simulink model "fxpdemo_sfun_user_prodsum"  (Simulink 7.6)
settings: Solver=FixedStepDiscrete  StartTime=0.0  StopTime=0.2  FixedStep=0.001  RelTol=1e-3
libraries: simulink x3
Description:
  | Fixed-Point S-Functions: Product and Sum
  | 
  | This model exercises a custom C language S-function written to compute a fixed-point
  | "product and sum" operation.  To see the source code for the S-function, use the right-click context menu to
  | select "Look Under Mask".  When the dialog box appears, press the Edit button.
settings Model: Creator=The MathWorks Inc.  ExtModeAutoUpdateStatusClock=off
settings DataIOCC: SignalLoggingName=sigsOut
settings OptimizationCC: InlineParams=on  InitFltsAndDblsToZero=on
settings DebuggingCC: SaveWithParameterizedLinksMsg=none  SignalResolutionControl=TryResolveAllWithWarning  SolverPrmCheckMsg=none  MultiTaskDSMMsg=warning  MultiTaskCondExecSysMsg=none  ParameterPrecisionLossMsg=none  StrictBusMsg=None
settings HardwareCC: TargetUnknown=on
settings RTWCC: GenerateReport=on  IncludeERTFirstTime=on
settings GRTTargetCC: TargetFcnLib=ansi_tfl_tmw.mat

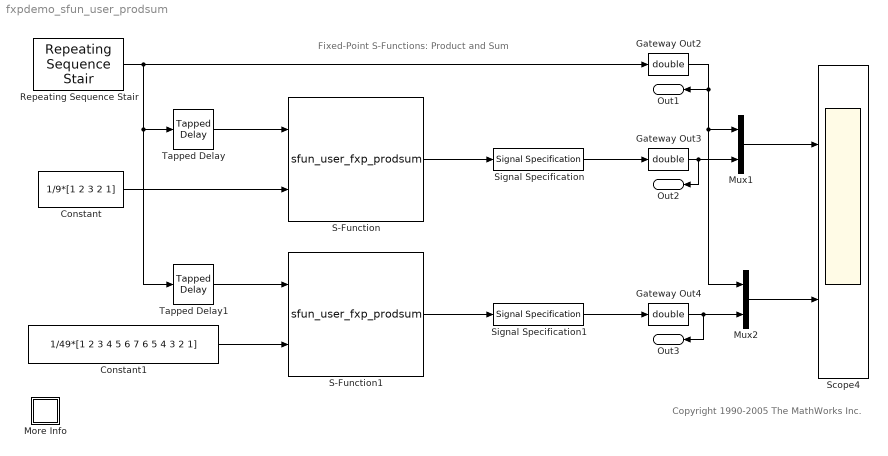
== system fxpdemo_sfun_user_prodsum ==
  note: Copyright 1990-2005 The MathWorks Inc.
  note: Fixed-Point S-Functions: Product and Sum
  Constant : Constant  Value=1/9*[1 2 3 2 1]  OutDataTypeStr=sfix(16)
  Constant1 : Constant  Value=1/49*[1 2 3 4 5 6 7 6 5 4 3 2 1]  OutDataTypeStr=fixdt(1,16,16)
  Gateway Out2 : DataTypeConversion  OutDataTypeStr=double  RndMeth=Zero
  Gateway Out3 : DataTypeConversion  OutDataTypeStr=double  RndMeth=Zero
  Gateway Out4 : DataTypeConversion  OutDataTypeStr=double  RndMeth=Zero
  More Info : Subsystem
      settings: OpenFcn=showdemo(bdroot(gcs))
      mask Display: disp('?')
  Mux1 : Mux  Inputs=2
  Mux2 : Mux  Inputs=2
  Repeating Sequence Stair : simulink/Sources/Repeating Sequence Stair  SystemSampleTime=-1  OutValues=5*sin(10*2*pi*(0:200)/200)  tsamp=-1  OutMin=[]  OutMax=[]  OutDataTypeStr=sfix(16)  OutputDataTypeScalingMode=Specify via dialog  OutDataType=sfix(16)  ConRadixGroup=Best Precision: Vector-wise  OutScaling=2^-12
  S-Function : S-Function  FunctionName=sfun_user_fxp_prodsum  EnableBusSupport=off
  S-Function1 : S-Function  FunctionName=sfun_user_fxp_prodsum  EnableBusSupport=off
  Scope4 : Scope  NumInputPorts=2
      settings: TimeRange=0.2  YMin=-5~-5  YMax=5~5  SaveName=ScopeData3
  Signal Specification : SignalSpecification  OutDataTypeStr=fixdt(1,16,12)
  Signal Specification1 : SignalSpecification  OutDataTypeStr=fixdt(1,16,10)
  Tapped Delay : simulink/Discrete/Tapped Delay  vinit=0.0  samptime=-1  NumDelays=5  DelayOrder=Oldest  includeCurrent=off
  Tapped Delay1 : simulink/Discrete/Tapped Delay  vinit=0.0  samptime=-1  NumDelays=13  DelayOrder=Oldest  includeCurrent=off
  Out1 : Outport
  Out2 : Outport  Port=2
  Out3 : Outport  Port=3
  wires:
  Mux1/1 -> Scope4/1
  Gateway Out3/1 -> Mux1/2, Out2/1
  S-Function/1 -> Signal Specification/1
  Constant/1 -> S-Function/2
  Tapped Delay/1 -> S-Function/1
  Signal Specification/1 -> Gateway Out3/1
  Mux2/1 -> Scope4/2
  Gateway Out4/1 -> Mux2/2, Out3/1
  S-Function1/1 -> Signal Specification1/1
  Signal Specification1/1 -> Gateway Out4/1
  Repeating Sequence Stair/1 -> Gateway Out2/1, Tapped Delay/1, Tapped Delay1/1
  Tapped Delay1/1 -> S-Function1/1
  Constant1/1 -> S-Function1/2
  Gateway Out2/1 -> Out1/1, Mux1/1, Mux2/1

== system fxpdemo_sfun_user_prodsum/More Info ==
